simulink model "CI"  (R2021b)
settings: Solver=VariableStepAuto  StartTime=0.0  StopTime=10.0  RelTol=1e-3
values from neighbouring files (symbols this model uses):
  clampingON = 0    [avaliaCI.m]    (also in compararAntiWindUps.m = 1)
  controlador = projetarControlador(planta)    [avaliaAS.m]    (also in avaliaBC1.m; avaliaBC2.m = projetarControladorPI(planta); avaliaCI.m; avaliaMalhaPura.m)
  planta = obterPlanta()    [avaliaAS.m]    (also in avaliaBC1.m; avaliaBC2.m; avaliaCI.m; avaliaMalhaPura.m)
settings Model: Creator=ariel  LastModifiedBy=ariel

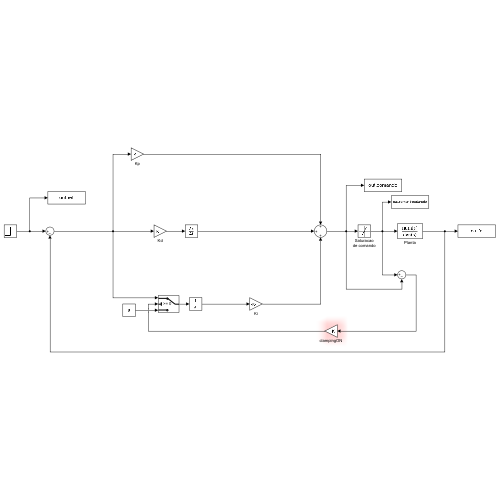
[thumbnail: Simulink's stored preview of the top-level diagram]
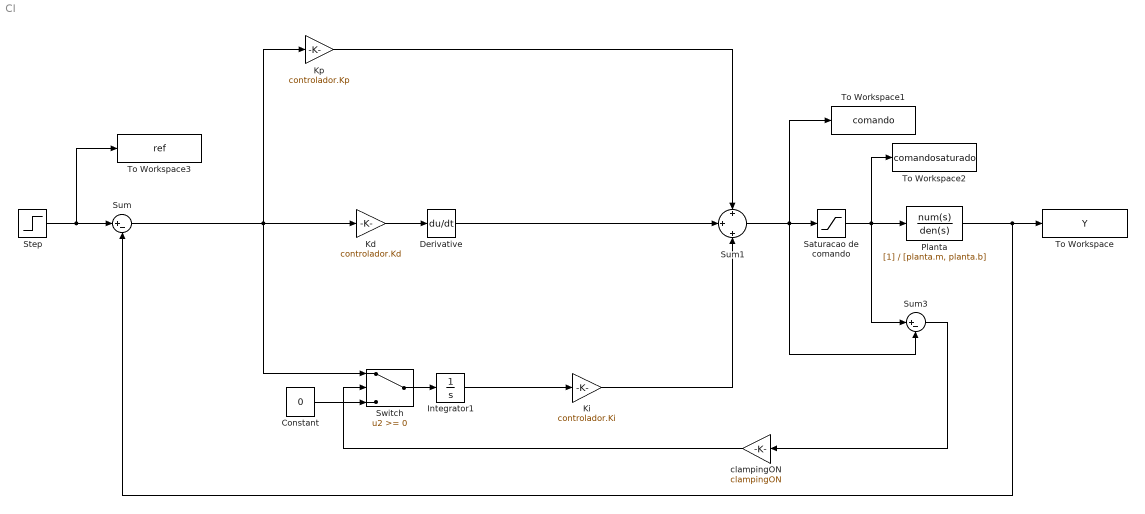
== system CI ==
  Constant : Constant  Value=0
  Derivative : Derivative
  Integrator1 : Integrator
  Kd : Gain  Gain=controlador.Kd
  Ki : Gain  Gain=controlador.Ki
  Kp : Gain  Gain=controlador.Kp
  Planta : TransferFcn  Denominator=[planta.m, planta.b]  ParameterTunability=Optimized
  Saturacao de comando : Saturate  UpperLimit=planta.comandoNominal  LowerLimit=-planta.comandoNominal
  Step : Step  SampleTime=0
  Sum : Sum  Inputs=|+-
  Sum1 : Sum  Inputs=+|+|+
  Sum3 : Sum  Inputs=|+-
  Switch : Switch
  To Workspace : ToWorkspace  VariableName=Y  SaveFormat=Structure With Time  SampleTime=-1
  To Workspace1 : ToWorkspace  VariableName=comando  SaveFormat=Structure With Time  SampleTime=-1
  To Workspace2 : ToWorkspace  VariableName=comandosaturado  SaveFormat=Structure With Time  SampleTime=-1
  To Workspace3 : ToWorkspace  VariableName=ref  SaveFormat=Structure With Time  SampleTime=-1
  clampingON : Gain  Gain=clampingON
  wires:
  Sum/1 -> Switch/1, Kd/1, Kp/1
  Ki/1 -> Sum1/3
  Kp/1 -> Sum1/1
  Kd/1 -> Derivative/1
  Derivative/1 -> Sum1/2
  Switch/1 -> Integrator1/1
  Integrator1/1 -> Ki/1
  Planta/1 -> To Workspace/1, Sum/2
  Sum1/1 -> Sum3/2, Saturacao de comando/1, To Workspace1/1
  Saturacao de comando/1 -> Sum3/1, To Workspace2/1, Planta/1
  Step/1 -> To Workspace3/1, Sum/1
  Constant/1 -> Switch/3
  Sum3/1 -> clampingON/1
  clampingON/1 -> Switch/2
